simulink model "ssc_simple_mechanical_system_Manuel"  (R2022a)
settings: Solver=ode1be  StartTime=0.0  StopTime=SimTime  FixedStep=Ts  MaxStep=0.2  RelTol=1e-3  AbsTol=1e-3  EnableMultiTasking=on
PreLoadFcn:
  | time_force = [0 0.2 0.34 3 3.22 6 6.2 10];
  | data_force = [0 0 12 12 -12 -12 0 0];
  | ts_force = timeseries(data_force,time_force,'Name','ts_force');
undefined symbols (not defined in the file): Switch, Ts
libraries: fl_lib x19, nesl_utility x3
CloseFcn:
  | clear simlog_ssc_simple_mechanical_system
  | 
  | clear time_force
  | clear data_force
  | clear ts_force
Description:
  | Simple Mechanical System
settings Model: Creator=The MathWorks, Inc.  LastModifiedBy=manue
settings SolverCC: AutoScaleAbsTol=off  AlgebraicLoopSolver=TrustRegion  MaxZcPerStep=1
settings DataIOCC: ExternalInput=ts_force  LimitDataPoints=on  LoadExternalInput=on  SaveFormat=Array  ReturnWorkspaceOutputs=off
settings OptimizationCC: ExpressionDepthLimit=2147483647  InitFltsAndDblsToZero=on  LifeSpan=inf
settings DebuggingCC: SaveWithParameterizedLinksMsg=none  UnderspecifiedInitializationDetection=Classic  MergeDetectMultiDrivingBlocksExec=none  SignalResolutionControl=TryResolveAllWithWarning  SolverPrmCheckMsg=warning  MultiTaskDSMMsg=warning  FcnCallInpInsideContextMsg=warning  UnconnectedInputMsg=warning  UnconnectedOutputMsg=warning  UnconnectedLineMsg=warning  AllowSymbolicDim=off  StateNameClashWarn=warning  PregeneratedLibrarySubsystemCodeDiagnostic=none  SFUnexpectedBacktrackingDiag=warning  SFNoUnconditionalDefaultTransitionDiag=warning  SFExecutionAtInitializationDiag=none  SFMachineParentedDataDiag=warning  ArithmeticOperatorsInVariantConditions=warning
settings HardwareCC: ProdBitPerPointer=32  ProdBitPerSizeT=32  ProdBitPerPtrDiffT=32  ProdLargestAtomicFloat=None  ProdIntDivRoundTo=Undefined  ProdEndianess=Unspecified  ProdWordSize=32  ProdHWDeviceType=32-bit Generic
settings ModelReferenceCC: PropagateSignalLabelsOutOfModel=off
settings SFSimCC: SimUseLocalCustomCode=off  CustomCodeUndefinedFunction=UseInterfaceOnly
settings RTWCC: RTWUseLocalCustomCode=off  DLArmComputeVersion=19.05
settings CodeAppCC: StateflowObjectComments=on
settings GRTTargetCC: TargetFcnLib=ansi_tfl_tmw.mat  TargetLangStandard=C89/C90 (ANSI)  CombineOutputUpdateFcns=off  GRTInterface=on
settings ConfigComp: CovMetricSettings=dw  CovSaveCumulativeToWorkspaceVar=on  CovSaveSingleToWorkspaceVar=on  CovExternalEMLEnable=off  CovSFcnEnable=off
settings SimscapeCC: SimscapeLogType=all  SimscapeLogSimulationStatistics=on  SimscapeLogName=simlog_ssc_simple_mechanical_system  SimscapeLogDataHistory=10000

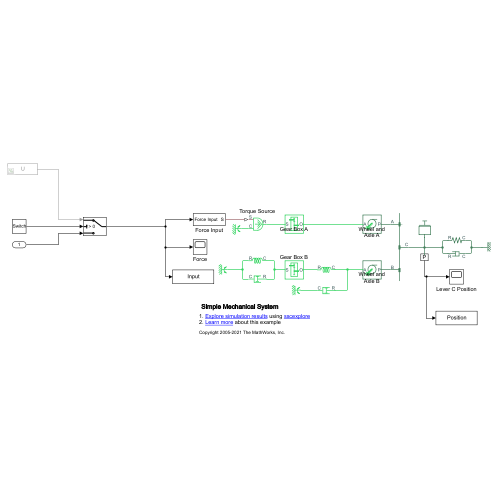
[thumbnail: Simulink's stored preview of the top-level diagram]
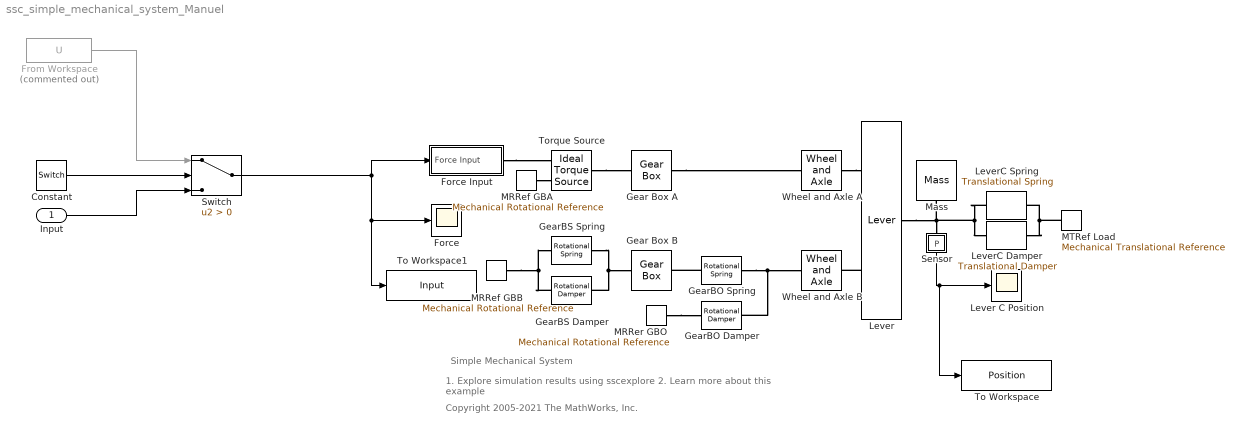
== system ssc_simple_mechanical_system_Manuel ==
  note: Simple Mechanical System
  note: 1. Explore simulation results using sscexplore
      | 2. Learn more about this example
  note: Copyright 2005-2021 The MathWorks, Inc.
  Input : Inport
  Constant : Constant  Value=Switch
  Force : Scope
  Force Input : Subsystem
  From Workspace : FromWorkspace  Commented=on  VariableName=U
  Gear Box A : fl_lib/Mechanical/Mechanisms/Gear Box  Tag=Factory Generic  ratio=5  t_in_specify=off  t_in_priority=High  t_in=0 N*m  t_in_nominal_specify=off  t_in_nominal_unit=N*m  t_in_nominal_value=1  t_out_specify=off  t_out_priority=High  t_out=0 N*m  t_out_nominal_specify=off  t_out_nominal_unit=N*m  t_out_nominal_value=1
      settings: SourceProductBaseCode=PW,SS,VE
  Gear Box B : fl_lib/Mechanical/Mechanisms/Gear Box  Tag=Factory Generic  ratio=2  t_in_specify=off  t_in_priority=High  t_in=0 N*m  t_in_nominal_specify=off  t_in_nominal_unit=N*m  t_in_nominal_value=1  t_out_specify=off  t_out_priority=High  t_out=0 N*m  t_out_nominal_specify=off  t_out_nominal_unit=N*m  t_out_nominal_value=1
      settings: SourceProductBaseCode=PW,SS,VE
  GearBO Damper : fl_lib/Mechanical/Rotational Elements/Rotational Damper  Tag=Factory Generic  D=0.0004 m*s*N/rad  w_specify=off  w_priority=High  w=0 rad/s  w_nominal_specify=off  w_nominal_unit=rad/s  w_nominal_value=1  t_specify=off  t_priority=High  t=0 N*m  t_nominal_specify=off  t_nominal_unit=N*m  t_nominal_value=1
      settings: SourceProductBaseCode=PW,SS,VE
  GearBO Spring : fl_lib/Mechanical/Rotational Elements/Rotational Spring  Tag=Factory Generic  spr_rate=100 N*m/rad  w_specify=off  w_priority=High  w=0 rad/s  w_nominal_specify=off  w_nominal_unit=rad/s  w_nominal_value=1  t_specify=off  t_priority=High  t=0 N*m  t_nominal_specify=off  t_nominal_unit=N*m  t_nominal_value=1  phi_specify=off  phi_priority=High  phi=0 rad  phi_nominal_specify=off  phi_nominal_unit=rad  phi_nominal_value=1
      settings: SourceProductBaseCode=PW,SS,VE
  GearBS Damper : fl_lib/Mechanical/Rotational Elements/Rotational Damper  Tag=Factory Generic  D=0.0006 m*s*N/rad  w_specify=off  w_priority=High  w=0 rad/s  w_nominal_specify=off  w_nominal_unit=rad/s  w_nominal_value=1  t_specify=off  t_priority=High  t=0 N*m  t_nominal_specify=off  t_nominal_unit=N*m  t_nominal_value=1
      settings: SourceProductBaseCode=PW,SS,VE
  GearBS Spring : fl_lib/Mechanical/Rotational Elements/Rotational Spring  Tag=Factory Generic  spr_rate=100 N*m/rad  w_specify=off  w_priority=High  w=0 rad/s  w_nominal_specify=off  w_nominal_unit=rad/s  w_nominal_value=1  t_specify=off  t_priority=High  t=0 N*m  t_nominal_specify=off  t_nominal_unit=N*m  t_nominal_value=1  phi_specify=off  phi_priority=High  phi=0 rad  phi_nominal_specify=off  phi_nominal_unit=rad  phi_nominal_value=1
      settings: SourceProductBaseCode=PW,SS,VE
  Lever : fl_lib/Mechanical/Mechanisms/Lever  Tag=Factory Generic  arm_AC=0.1 m  arm_BC=0.1 m  f_A_specify=off  f_A_priority=High  f_A=0 N  f_A_nominal_specify=off  f_A_nominal_unit=N  f_A_nominal_value=1  f_B_specify=off  f_B_priority=High  f_B=0 N  f_B_nominal_specify=off  f_B_nominal_unit=N  f_B_nominal_value=1  f_C_specify=off  f_C_priority=High  f_C=0 N  f_C_nominal_specify=off  f_C_nominal_unit=N  f_C_nominal_value=1
      settings: SourceProductBaseCode=PW,SS,VE  InternalSimscapePortConfiguration="{\"Bottom\":[],\"Left\":[{\"id\":\"A\",\"label\":\"A\",\"type\":\"foundation.mechanical.translational.translational\"},{\"id\":\"B\",\"label\":\"B\",\"type\":\"foundation.mechanical.translational.translational\"}],\"Right\":[{\"id\":\"C\",\"label\":\"C\",\"type\":\"foundation.mechanical.translational.translational\"}],\"Top\":[]}"
  Lever C Position : Scope
  LeverC Damper : fl_lib/Mechanical/Translational Elements/Translational Damper  Tag=Factory Generic  D=64 s*N/m  v_specify=off  v_priority=High  v=0 m/s  v_nominal_specify=off  v_nominal_unit=m/s  v_nominal_value=1  f_specify=off  f_priority=High  f=0 N  f_nominal_specify=off  f_nominal_unit=N  f_nominal_value=1
      settings: SourceProductBaseCode=PW,SS,VE
  LeverC Spring : fl_lib/Mechanical/Translational Elements/Translational Spring  Tag=Factory Generic  spr_rate=10000 N/m  v_specify=off  v_priority=High  v=0 m/s  v_nominal_specify=off  v_nominal_unit=m/s  v_nominal_value=1  f_specify=off  f_priority=High  f=0 N  f_nominal_specify=off  f_nominal_unit=N  f_nominal_value=1  x_specify=off  x_priority=High  x=0 m  x_nominal_specify=off  x_nominal_unit=m  x_nominal_value=1
      settings: SourceProductBaseCode=PW,SS,VE
  MRRef GBA : fl_lib/Mechanical/Rotational Elements/Mechanical Rotational Reference  Tag=Factory Generic
      settings: SourceProductBaseCode=PW,SS,VE
  MRRef GBB : fl_lib/Mechanical/Rotational Elements/Mechanical Rotational Reference  Tag=Factory Generic
      settings: SourceProductBaseCode=PW,SS,VE
  MRRer GBO : fl_lib/Mechanical/Rotational Elements/Mechanical Rotational Reference  Tag=Factory Generic
      settings: SourceProductBaseCode=PW,SS,VE
  MTRef Load : fl_lib/Mechanical/Translational Elements/Mechanical Translational Reference  Tag=Factory Generic
      settings: SourceProductBaseCode=PW,SS,VE
  Mass : fl_lib/Mechanical/Translational Elements/Mass  Tag=Factory Generic  mass=12 kg  num_ports=foundation.enum.numPorts2.one  v_specify=off  v_priority=High  v=0 m/s  v_nominal_specify=off  v_nominal_unit=m/s  v_nominal_value=1  f_specify=off  f_priority=High  f=0 N  f_nominal_specify=off  f_nominal_unit=N  f_nominal_value=1
      settings: SourceProductBaseCode=PW,SS,VE
  Sensor : Subsystem
      mask Display: disp('P')
  Switch : Switch  Criteria=u2 > Threshold  SaturateOnIntegerOverflow=off  InputSameDT=off
  To Workspace : ToWorkspace  VariableName=Position  SampleTime=Ts
  To Workspace1 : ToWorkspace  VariableName=Input  SampleTime=Ts
  Torque Source : fl_lib/Mechanical/Mechanical Sources/Ideal Torque Source  Tag=Factory Generic
      settings: SourceProductBaseCode=PW,SS,VE
  Wheel and Axle A : fl_lib/Mechanical/Mechanisms/Wheel and Axle  Tag=Factory Generic  R=0.05 m  or=1  t_specify=off  t_priority=High  t=0 N*m  t_nominal_specify=off  t_nominal_unit=N*m  t_nominal_value=1  f_specify=off  f_priority=High  f=0 N  f_nominal_specify=off  f_nominal_unit=N  f_nominal_value=1
      settings: SourceProductBaseCode=PW,SS,VE
  Wheel and Axle B : fl_lib/Mechanical/Mechanisms/Wheel and Axle  Tag=Factory Generic  R=0.08 m  or=1  t_specify=off  t_priority=High  t=0 N*m  t_nominal_specify=off  t_nominal_unit=N*m  t_nominal_value=1  f_specify=off  f_priority=High  f=0 N  f_nominal_specify=off  f_nominal_unit=N  f_nominal_value=1
      settings: SourceProductBaseCode=PW,SS,VE
  wires:
  Sensor/1(P) -> To Workspace/1, Lever C Position/1
  Switch/1 -> Force Input/1(Force Input), To Workspace1/1, Force/1
  Input/1 -> Switch/3
  Constant/1 -> Switch/2
  From Workspace/1 -> Switch/1
  connections:
  Torque Source/LConn1 -- Gear Box A/LConn1
  Gear Box A/RConn1 -- Wheel and Axle A/LConn1
  Wheel and Axle A/RConn1 -- Lever/LConn1
  Lever/LConn2 -- Wheel and Axle B/RConn1
  LeverC Spring/LConn1 -- Lever/RConn1 -- Sensor/LConn1 -- Mass/LConn1 -- LeverC Damper/LConn1
  MTRef Load/LConn1 -- LeverC Damper/RConn1 -- LeverC Spring/RConn1
  MRRef GBA/LConn1 -- Torque Source/RConn2
  GearBO Spring/LConn1 -- Gear Box B/RConn1
  MRRer GBO/LConn1 -- GearBO Damper/RConn1
  MRRef GBB/LConn1 -- GearBS Damper/RConn1 -- GearBS Spring/LConn1
  GearBS Spring/RConn1 -- GearBS Damper/LConn1 -- Gear Box B/LConn1
  GearBO Spring/RConn1 -- Wheel and Axle B/LConn1 -- GearBO Damper/LConn1
  Force Input/RConn1 -- Torque Source/RConn1

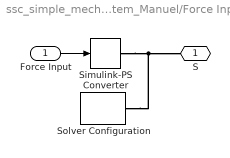
== system ssc_simple_mechanical_system_Manuel/Force Input ==
  Force Input : Inport
  Simulink-PS Converter : nesl_utility/Simulink-PS Converter  PhysicalDomain=network_engine_domain  SubClassName=ps_input  LeftPortType=input  RightPortType=output  PseudoPeriodic=off  Frequencies=[]  NoiseDistribution=none  NoiseParameters=[]  Unit=1  AffineConversion=off  FilteringAndDerivatives=zero  SimscapeFilterOrder=1  InputFilterTimeConstant=.001  UdotUserProvided=[]
      settings: SourceProductBaseCode=SS,PW,VE
  Solver Configuration : nesl_utility/Solver Configuration  PhysicalDomain=network_engine_domain  SubClassName=solver  LeftPortType=input  RightPortType=generic  Tones=[]  Harmonics=[]  SimulateNoise=off  Profile=off  UseLocalSampling=off  EnableSwitchedLinearOptims=on  FrequencyDomain=off  UseCCode=off  RelTol=0.001  AbsTol=1e-06  MinStep=1e-09  ToWorkspace=off  RevertToSquareIcSolve=off  NumHomotopyIterations=100  PhasorMode=off  PhasorModeNumHarmonics=1  IndexReductionMethod=DerivativeReplacement  DoDC=off  ResidualTolerance=1e-9  UseLocalSolver=on  LocalSolverChoice=NE_BACKWARD_EULER_ADVANCER  LocalSolverSampleTime=Ts  DoFixedCost=on  MaxNonlinIter=3  MaxModeIter=2  ComputeImpulses=off  ImpulseIterations=2  LinearAlgebra=auto  LinearAlgebraNumThread=0  EquationFormulation=NE_TIME_EF  DelaysMemoryBudget=1024  AutomaticFiltering=on  FilteringTimeConstant=0.001  PartitionStorageMethod=AS_NEEDED  PartitionMemoryBudget=1024  PartitionMethod=FAST
      settings: SourceProductBaseCode=SS,PW,VE
  S : PMIOPort  Side=Right
  wires:
  Force Input/1 -> Simulink-PS Converter/1
  connections:
  Simulink-PS Converter/RConn1 -- Solver Configuration/RConn1 -- S/RConn1

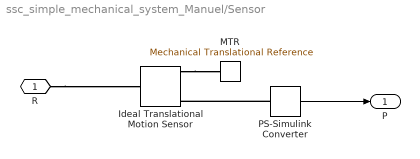
== system ssc_simple_mechanical_system_Manuel/Sensor ==
  Ideal Translational Motion Sensor : fl_lib/Mechanical/Mechanical Sensors/Ideal Translational Motion Sensor  Tag=Factory Generic  offset=0 m
      settings: SourceProductBaseCode=PW,SS,VE
  MTR : fl_lib/Mechanical/Translational Elements/Mechanical Translational Reference  Tag=Factory Generic
      settings: SourceProductBaseCode=PW,SS,VE
  PS-Simulink Converter : nesl_utility/PS-Simulink Converter  PhysicalDomain=network_engine_domain  SubClassName=ps_output  LeftPortType=input  RightPortType=output  PseudoPeriodic=off  Frequencies=[]  VectorFormat=1-D array  Unit=1  AffineConversion=off
      settings: SourceProductBaseCode=SS,PW,VE
  R : PMIOPort  Side=Left
  P : Outport  VectorParamsAs1DForOutWhenUnconnected=off
  wires:
  PS-Simulink Converter/1 -> P/1
  connections:
  Ideal Translational Motion Sensor/RConn1 -- MTR/LConn1
  PS-Simulink Converter/LConn1 -- Ideal Translational Motion Sensor/RConn3
  R/RConn1 -- Ideal Translational Motion Sensor/LConn1
